simulink model "pathFollowing"  (R2017a)
settings: Solver=FixedStepDiscrete  StartTime=0.0  StopTime=Inf  FixedStep=0.1  RelTol=1e-3  EnableMultiTasking=on
model workspace (MAT data in the model file):
  SL_ROS_VariableLengthArrays_MaxSizes.CommonInfo.ArrayTruncateAction = 'EmitWarning'
  SL_ROS_VariableLengthArrays_MaxSizes.MsgTypeMap = containers.Map
  SL_ROS_VariableLengthArrays_MaxSizes.MsgTypeMap.serialization.keys = {'sensor_msgs/Image', 'sensor_msgs/LaserScan'}
  SL_ROS_VariableLengthArrays_MaxSizes.MsgTypeMap.serialization.values{1}(1).PropertyName = 'Data'
  SL_ROS_VariableLengthArrays_MaxSizes.MsgTypeMap.serialization.values{1}(1).DataType = 'uint8'
  SL_ROS_VariableLengthArrays_MaxSizes.MsgTypeMap.serialization.values{1}(1).MaxLength = 691200
  SL_ROS_VariableLengthArrays_MaxSizes.MsgTypeMap.serialization.values{1}(2).PropertyName = 'Encoding'
  SL_ROS_VariableLengthArrays_MaxSizes.MsgTypeMap.serialization.values{1}(2).DataType = 'uint8'
  SL_ROS_VariableLengthArrays_MaxSizes.MsgTypeMap.serialization.values{1}(2).MaxLength = 128
  SL_ROS_VariableLengthArrays_MaxSizes.MsgTypeMap.serialization.values{2}(1).PropertyName = 'Intensities'
  SL_ROS_VariableLengthArrays_MaxSizes.MsgTypeMap.serialization.values{2}(1).DataType = 'single'
  SL_ROS_VariableLengthArrays_MaxSizes.MsgTypeMap.serialization.values{2}(1).MaxLength = 1080
  SL_ROS_VariableLengthArrays_MaxSizes.MsgTypeMap.serialization.values{2}(2).PropertyName = 'Ranges'
  SL_ROS_VariableLengthArrays_MaxSizes.MsgTypeMap.serialization.values{2}(2).DataType = 'single'
  SL_ROS_VariableLengthArrays_MaxSizes.MsgTypeMap.serialization.values{2}(2).MaxLength = 1080
  SL_ROS_VariableLengthArrays_MaxSizes.MsgTypeMap.serialization.uniformity = 0
  SL_ROS_VariableLengthArrays_MaxSizes.MsgTypeMap.serialization.keyType = 'char'
  SL_ROS_VariableLengthArrays_MaxSizes.MsgTypeMap.serialization.valueType = 'any'
undefined symbols (not defined in the file): Angular, gray, Linear
libraries: robotlib x6, robotalgslib x1, aerolibanimutils x1, simulink x1
settings Model: Creator=The MathWorks, Inc.  LastModifiedBy=jcassett
settings DataIOCC: LimitDataPoints=on  SaveFormat=Array
settings OptimizationCC: LifeSpan=Inf  MaxStackSize=64
settings DebuggingCC: SolverPrmCheckMsg=warning  SFUnexpectedBacktrackingDiag=warning  SFNoUnconditionalDefaultTransitionDiag=warning  SFExecutionAtInitializationDiag=none
settings HardwareCC: ProdBitPerPointer=32  ProdBitPerSizeT=32  ProdBitPerPtrDiffT=32  ProdLargestAtomicFloat=None  ProdIntDivRoundTo=Undefined  ProdEndianess=Unspecified  ProdWordSize=32  ProdHWDeviceType=Generic->Unspecified (assume 32-bit Generic)  UseEmbeddedCoderFeatures=off
settings ModelReferenceCC: PropagateSignalLabelsOutOfModel=off
settings RTWCC: SystemTargetFile=ert.tlc  HardwareBoard=Robot Operating System (ROS)  TLCOptions=-aInlineSetEventsForThisBaseRateFcn=TLC_FALSE -aSuppressMultiTaskScheduler=TLC_FALSE -aRateBasedStepFcn=0  TemplateMakefile=ert_default_tmf  Description=Embedded Coder  Toolchain=Catkin  TargetLang=C++
settings ERTTargetCC: MultiwordLength=2048  ERTCustomFileBanners=off  SupportContinuousTime=on  SupportNonInlinedSFcns=on  RemoveResetFunc=off  SupportVariableSizeSignals=on  ModelStepFunctionPrototypeControlCompliant=off  ConvertIfToSwitch=off  SuppressUnreachableDefaultCases=off
settings ConfigComp: CovMetricSettings=dw  CovHtmlReporting=on  CovSaveCumulativeToWorkspaceVar=on  CovSaveSingleToWorkspaceVar=on  CovExternalEMLEnable=off  CovSFcnEnable=off

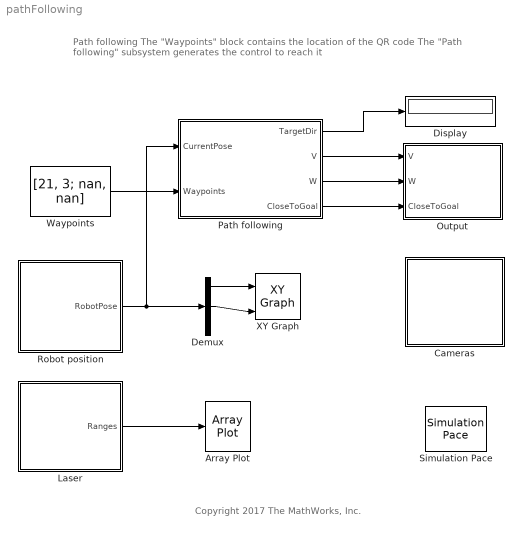
== system pathFollowing ==
  note: Path following
      | The "Waypoints" block contains the location of the QR code
      | The "Path following" subsystem generates the control to reach it
  note: Copyright 2017 The MathWorks, Inc.
  Array Plot : ArrayPlot
  Cameras : Subsystem
  Demux : Demux  Outputs=3
  Display : Display
  Laser : Subsystem
  Output : Subsystem
  Path following : Subsystem
  Robot position : Subsystem
  Simulation Pace : aerolibanimutils/Simulation Pace  SimulationPace=1  SleepMode=MATLAB Thread  OutputPaceError=off  SampleTime=-1
  Waypoints : Constant  Value=[21, 3; nan, nan]  OutDataTypeStr=double
  XY Graph : simulink/Sinks/XY Graph  xmin=-10  xmax=30  ymin=-10  ymax=10  st=-1
  wires:
  Robot position/1(RobotPose) -> Path following/1(CurrentPose), Demux/1
  Demux/1 -> XY Graph/1
  Demux/2 -> XY Graph/2
  Laser/1(Ranges) -> Array Plot/1
  Waypoints/1 -> Path following/2(Waypoints)
  Path following/2(V) -> Output/1(V)
  Path following/4(CloseToGoal) -> Output/3(CloseToGoal)
  Path following/3(W) -> Output/2(W)
  Path following/1(TargetDir) -> Display/1

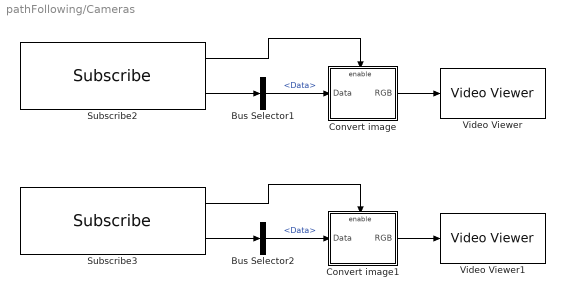
== system pathFollowing/Cameras ==
  Bus Selector1 : BusSelector  DialogController=Simulink.DDGSource_BusSelector  OutputSignals=Data
  Bus Selector2 : BusSelector  DialogController=Simulink.DDGSource_BusSelector  OutputSignals=Data
  Convert image : Subsystem
  Convert image1 : Subsystem
  Subscribe2 : robotlib/Subscribe  SourceLibraryInfo=This block requires Robotics System Toolbox  topicSource=Select from ROS network  topic=/quadrotor_1/front/image_raw  messageType=sensor_msgs/Image  sampleTime=-1  messageQueueLength=51
      settings: SourceProductBaseCode=RO
  Subscribe3 : robotlib/Subscribe  SourceLibraryInfo=This block requires Robotics System Toolbox  topicSource=Select from ROS network  topic=/quadrotor_1/bottom/image_raw  messageType=sensor_msgs/Image  sampleTime=-1  messageQueueLength=51
      settings: SourceProductBaseCode=RO
  Video Viewer : VideoViewer  colormapValue=gray(256)  FigPos=[1022.09090909091 508.545454545455 609.163636363637 376.145454545455]
  Video Viewer1 : VideoViewer  colormapValue=gray(256)  FigPos=[1013.36363636364 1003.38181818182 609.163636363636 376.145454545455]
  wires:
  Subscribe2/1 -> Convert image/Enable
  Convert image1/1(RGB) -> Video Viewer1/1
  Subscribe3/2 -> Bus Selector2/1
  Subscribe2/2 -> Bus Selector1/1
  Bus Selector1/1 -> Convert image/1(Data)  "<Data>"
  Bus Selector2/1 -> Convert image1/1(Data)  "<Data>"
  Subscribe3/1 -> Convert image1/Enable
  Convert image/1(RGB) -> Video Viewer/1

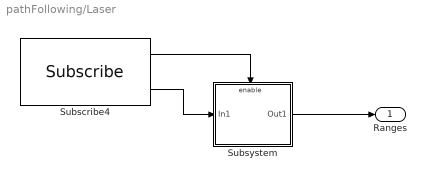
== system pathFollowing/Laser ==
  Subscribe4 : robotlib/Subscribe  SourceLibraryInfo=This block requires Robotics System Toolbox  topicSource=Select from ROS network  topic=/quadrotor_1/scan  messageType=sensor_msgs/LaserScan  sampleTime=-1  messageQueueLength=51
      settings: SourceProductBaseCode=RO
  Subsystem : Subsystem
  Ranges : Outport
  wires:
  Subsystem/1(Out1) -> Ranges/1
  Subscribe4/2 -> Subsystem/1(In1)
  Subscribe4/1 -> Subsystem/Enable

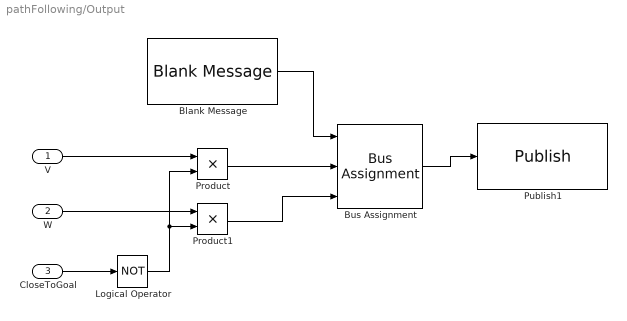
== system pathFollowing/Output ==
  V : Inport
  W : Inport  Port=2
  CloseToGoal : Inport  Port=3
  Blank Message : robotlib/Blank Message  SourceLibraryInfo=This block requires Robotics System Toolbox  messageType=geometry_msgs/Twist  SampleTime=0
      settings: SourceProductBaseCode=RO
  Bus Assignment : BusAssignment  DialogController=Simulink.DDGSource_BusAssignment  AssignedSignals=Linear.X,Angular.Z
  Logical Operator : Logic  Operator=NOT  AllPortsSameDT=off  OutDataTypeStr=boolean
  Product : Product
  Product1 : Product
  Publish1 : robotlib/Publish  SourceLibraryInfo=This block requires Robotics System Toolbox  topicSource=Select from ROS network  topic=/quadrotor_1/cmd_vel  messageType=geometry_msgs/Twist  messageQueueLength=105
      settings: SourceProductBaseCode=RO
  wires:
  Bus Assignment/1 -> Publish1/1
  Blank Message/1 -> Bus Assignment/1
  Logical Operator/1 -> Product1/2, Product/2
  Product1/1 -> Bus Assignment/3
  CloseToGoal/1 -> Logical Operator/1
  Product/1 -> Bus Assignment/2
  V/1 -> Product/1
  W/1 -> Product1/1

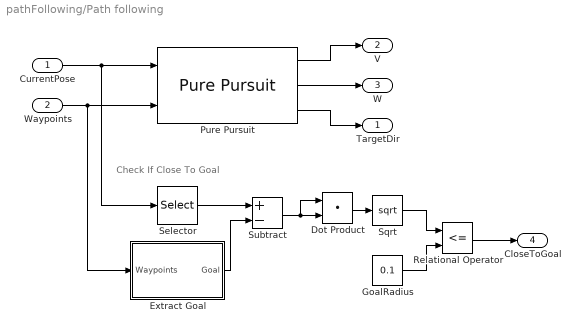
== system pathFollowing/Path following ==
  note: Check If Close To Goal
  CurrentPose : Inport
  Waypoints : Inport  Port=2
  " Extract Goal" : MATLAB Function  TreatAsAtomicUnit=on
  Dot Product : DotProduct  InputSameDT=on  OutDataTypeStr=Inherit: Inherit via internal rule
  GoalRadius : Constant  Value=0.1
  Pure Pursuit : robotalgslib/Pure Pursuit  DesiredLinearVelocity=0.3  MaxAngularVelocity=1.0  LookaheadDistance=2.0  TargetDirPort=on  SimulateUsing=Code generation
      settings: SourceProductName=Robotics System Toolbox  SourceProductBaseCode=RO
  Relational Operator : RelationalOperator  Operator=<=  OutDataTypeStr=boolean  RndMeth=Simplest
  Selector : Selector  InputPortWidth=3  IndexOptions=Index vector (dialog)  Indices=[1 2]  OutputSizes=1
  Sqrt : Sqrt  SaturateOnIntegerOverflow=on
  Subtract : Sum  Inputs=+-
  TargetDir : Outport
  V : Outport  Port=2
  W : Outport  Port=3
  CloseToGoal : Outport  Port=4
  wires:
  Pure Pursuit/3 -> TargetDir/1
  Pure Pursuit/2 -> W/1
  Pure Pursuit/1 -> V/1
  " Extract Goal"/1(Goal) -> Subtract/2
  Waypoints/1 -> " Extract Goal"/1(Waypoints), Pure Pursuit/2
  CurrentPose/1 -> Selector/1, Pure Pursuit/1
  Relational Operator/1 -> CloseToGoal/1
  GoalRadius/1 -> Relational Operator/2
  Selector/1 -> Subtract/1
  Dot Product/1 -> Sqrt/1
  Sqrt/1 -> Relational Operator/1
  Subtract/1 -> Dot Product/1, Dot Product/2

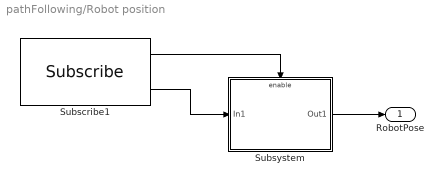
== system pathFollowing/Robot position ==
  Subscribe1 : robotlib/Subscribe  SourceLibraryInfo=This block requires Robotics System Toolbox  topicSource=Select from ROS network  topic=/quadrotor_1/ground_truth/state  messageType=nav_msgs/Odometry  sampleTime=-1  messageQueueLength=51
      settings: SourceProductBaseCode=RO
  Subsystem : Subsystem
  RobotPose : Outport
  wires:
  Subscribe1/1 -> Subsystem/Enable
  Subscribe1/2 -> Subsystem/1(In1)
  Subsystem/1(Out1) -> RobotPose/1

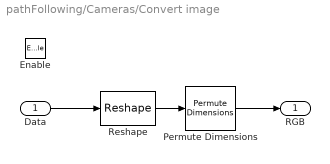
== system pathFollowing/Cameras/Convert image ==
  Data : Inport
  Enable : EnablePort
  Permute Dimensions : PermuteDimensions  Order=[3 2 1]
  Reshape : Reshape  OutputDimensionality=Customize  OutputDimensions=[3 640 360]
  RGB : Outport
  wires:
  Permute Dimensions/1 -> RGB/1
  Reshape/1 -> Permute Dimensions/1
  Data/1 -> Reshape/1

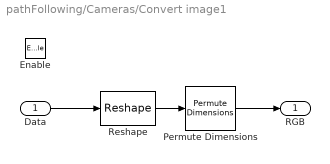
== system pathFollowing/Cameras/Convert image1 ==
  Data : Inport
  Enable : EnablePort
  Permute Dimensions : PermuteDimensions  Order=[3 2 1]
  Reshape : Reshape  OutputDimensionality=Customize  OutputDimensions=[3 640 360]
  RGB : Outport
  wires:
  Permute Dimensions/1 -> RGB/1
  Reshape/1 -> Permute Dimensions/1
  Data/1 -> Reshape/1

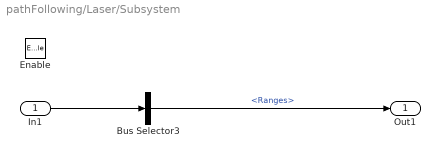
== system pathFollowing/Laser/Subsystem ==
  In1 : Inport
  Enable : EnablePort
  Bus Selector3 : BusSelector  DialogController=Simulink.DDGSource_BusSelector  OutputSignals=Ranges
  Out1 : Outport
  wires:
  Bus Selector3/1 -> Out1/1  "<Ranges>"
  In1/1 -> Bus Selector3/1

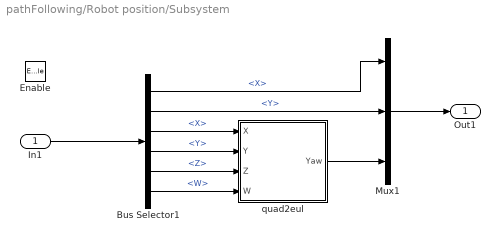
== system pathFollowing/Robot position/Subsystem ==
  In1 : Inport
  Enable : EnablePort
  Bus Selector1 : BusSelector  OutputSignals=Pose.Pose.Position.X,Pose.Pose.Position.Y,Pose.Pose.Orientation.X,Pose.Pose.Orientation.Y,Pose.Pose.Orientation.Z,Pose.Pose.Orientation.W
  Mux1 : Mux  Inputs=3
  quad2eul : MATLAB Function  TreatAsAtomicUnit=on
  Out1 : Outport
  wires:
  Bus Selector1/5 -> quad2eul/3(Z)  "<Z>"
  Bus Selector1/4 -> quad2eul/2(Y)  "<Y>"
  Bus Selector1/3 -> quad2eul/1(X)  "<X>"
  Bus Selector1/2 -> Mux1/2  "<Y>"
  quad2eul/1(Yaw) -> Mux1/3
  Mux1/1 -> Out1/1
  Bus Selector1/6 -> quad2eul/4(W)  "<W>"
  Bus Selector1/1 -> Mux1/1  "<X>"
  In1/1 -> Bus Selector1/1

== matlab function pathFollowing/Robot position/Subsystem/quad2eul ==
  data: X input; Yaw output; Y input; Z input; W input
function Yaw = quat2eulBlk(X, Y, Z, W)
%#codegen

eularAngles = quat2eul([W, X, Y, Z]);
Yaw = eularAngles(1);

== matlab function pathFollowing/Path following/ Extract Goal ==
  data: Waypoints input; Goal output
function Goal = extractGoal(Waypoints)
%#codegen
b = isnan(Waypoints);
[rows,~] = find(b);
ridx = setdiff(1:size(Waypoints,1), sort(rows));
Goal = [Waypoints(ridx(end), 1) Waypoints(ridx(end), 2)];
